simulink library "SDTlibV1"  (R2025b)
settings: Solver=VariableStepAuto  StartTime=0.0  StopTime=10.0  RelTol=1e-3
PreLoadFcn:
  | addpath(genpath('SDTfct'));
values from neighbouring files (symbols this model uses):
  pass = ra2DCMi(blk.ra)    [view_SDTlib_model.m]
undefined symbols (not defined in the file or in its folder): CMG, DAP0, DPa0, FSM, Ignew, InvDyn, InvDynAug, Jr, KIN, kinematic_model, LS, Mdyn, mnew, mp, OGnew, PMA, ra_norm, RWS, sig4, uls, ureal, uss, uw, XI
libraries: RCTblocks x470, $bdroot x4
(part 2 of 10)

== system SDTlibV1/6 dof mechanisms ==
  1 port spinning wheel : Subsystem  mask(One-port spinning wheel (6x18)){ra=[0;0;1], m=0.5, Iw=1, Ir=1/2, OG=[0;0;1], OP=[0;0;0], Omega=ureal('Omega',1000,'Range',[0 2000])}
      mask prompts: ra "Wheel axis (3x1 vector)"; m "Wheel mass (Kg)"; Iw "Wheel axial Inertia  (at G, Kgm^2)"; Ir "Wheel radial inertia (at G, Kgm^2)"; OG "OG (3x1 vector, m)"; OP "OP (3x1 vector, m)"; Omega "spinning rate (rd/s)"
      mask help:
      | Dynamic model of an onboard angular momentum (spinning wheel) at point P (connection point with a parent body):
      | 6x18 transfer between motion vector  at P and wrench applied by this body at P.
      | 0: the reference point
      | G: the center of the wheel
      | P: the connection point
      |
      | All parameters are expressed in the (inherit) body frame.
      | Only the spinning rate can be an uncertain parameter declared with "ureal"
      mask init:
      | pass=ra2DCMi(ra);
      | Tau_GP=kinematic_model(OG,OP);
      mask Help: web('DocMomentum.html','-browser','-browser')
      mask DialogControl ParameterGroupVar Prompt: Main parameters
      mask Display:
      | disp('One-port\n angular momemtum\n (6x18)')
      | port_label('input', 1, 'm')
      | port_label('output', 1, 'Wbody/.')
  2 phase stepper motor (r): TITOP model : Subsystem  mask(Stepper motor (in the load frame)){ra=[0;-1;0], z=90, p=4, n=8, I=0.17, Jr=1.1e-4, Km=4.44, C0=13e-4}
      mask prompts: ra "Direction of the joint in the local frame (3x1 vector)"; z "Rotor teeth number (integer)"; p "Stator beat number (integer)"; n "Subdivision number (integer)"; I "Current amplititude (A)"; Jr "Rotor inertia (Kg m^2)"; Km "Motor torque constant (Nm/A/rd)"; C0 "Viscous damping (Nms/rd)"
      mask help:
      | This block implement the TITOP model of a 2 phase stepper motor.
      | The direction of the revolute joint (3x1 vector) is respect with the load frame.
      |
      | LINEAR MODEL: valid around  the initial angular configuration
      | (joint angle in rad).
      |
      | Rotor inertia cannot be 0.
      mask init:
      | gam=2*pi/p/n;
      | K0=Km*I*z;
      | ra=[ra(1);ra(2);ra(3)]/norm(ra);
      | pass=[null(ra') ra];
      mask Help: web('DocStepperMotor_joly.html','-browser','-browser')
      mask Display:
      | disp('Stepper motor\n TITOP model')
      | port_label('input', 1, 'W./r')
      | port_label('output', 1, 'm_out')
      | port_label('input', 2, 'm_in')
      | port_label('output', 2, 'Wr/.')
      | port_label('input', 3, '\mu-step (int)','interpreter','tex')
      | port_label('output', 3, 'm_\theta','interpreter','tex')
  Gear box (G): TITOP model TO BE CHECKED!! : Subsystem  mask(Gear box){ra=[0;-1;0], N=-184, Jo=0.0001, Ji=0, Kg=9600, Cg=0.1}
      mask prompts: ra "Direction of the joint in the local frame (3x1 vector)"; N "Gear Box ratio"; Jo "Output shaft inertia (Kg.m^2)"; Ji "Input shaft inerta (Kg.m^2)"; Kg "Stiffness (output shaft Nm/rd)"; Cg "Viscous damping (output shaft Nms/rd)"
      mask help:
      | This block implement the TITOP model of a co-axial gearbox.
      | The direction of the gearbox axis (3x1 vector) is respect with the load frame)
      |
      | LINEAR MODEL: valid around delta_theta_o=0
      | (delta_theta_o is the geabox deflection in rad, seen from the output shaft).
      |
      | Output shaft inertia cannot be 0. If unknown, It is recommended to enter a small value (1/1000) w.r.t. the load (Kgm^2) connected on the output port.
      mask init:
      | ra=[ra(1);ra(2);ra(3)]/norm(ra);
      | pass=[null(ra') ra];
      mask Help: web('DocGearBox_joly.html','-browser','-browser')
      mask Display:
      | disp('Gear Box\n TITOP model')
      | port_label('input', 1, 'W./Go')
      | port_label('output', 1, 'm_out')
      | port_label('input', 2, 'm_in')
      | port_label('output', 2, 'WGi/.')
      | port_label('input', 3, 'Harm. pert. (Nm)')
      | port_label('output', 3, 'm_{\theta_o}','interpreter','tex')
  "Local Spring-Damper system " : Subsystem  mask(Local stiffness damper){K_O=diag([1 1 1 2 2 2]), D_O=diag([10 10 10 20 20 20]), OP=[0;0;0], OC=[0;0;0]}
      mask prompts: K_O "6x6 stiffness matrix at point O (N/m, Nm/rad)"; D_O "6x6 damping matrix  at point O (Ns/m, Nms/rad)"; OP "OP (3x1 vector (m)"; OC "OC (3x1 vector  (m)"
      mask help:
      | 12x36 TITOP model of a massless spring-damper system between:
      |   * the 2 motion vectors (inputs)  at the parent port (point P) and the child port (point C).
      |   *  the outside wrench applied to the spring-damper  at point C and the wrench applied by the spring-damper to outside at point P.
      | The model is expressed In the inherit reference frame.
      |
      | All the parameters can be declared as uncertain parameters (ureal(...)).
      mask init:
      | TAU_OC=kinematic_model([0;0;0],OC);
      | TAU_OP=kinematic_model([0;0;0],OP);
      mask Help: web('Doc_6DOFs_spring_damper.html','-browser','-browser')
      mask DialogControl ParameterGroupVar Prompt: Main parameters
      mask Display:
      | disp('Local\n spring-damper\n')
      | 
      | port_label('input', 1,'m_C')
      | port_label('output',1,'W./s,C')
      | port_label('input', 2,'m_P')
      | port_label('output',2,'Ws/.,P')
  PMA : Subsystem  mask(Proof mass actuator){Mc=0.5, IatG=diag([5e-3;5e-3;1.6e-4]), OG=[0;0;0.05], OP=[0;0;0], v=[0;0;1], mp=0.1, k=10, d=1.4}
      mask prompts: Mc "PMA total mass (Kg)"; IatG "PMA total inertia at G (Kgm^2)"; OG "OG (3x1 vector, m)"; OP "OP (3x1 vector, m)"; v "v (3x1 vector)"; mp "Proof mass (Kg)"; k "Stiffness (N/m)"; d "Damper (Ns/m)"
      mask help:
      | 7x19 dynamic model of PMA (Proof Mass Actuator) located at point P (connection point with the hub):
      |   * 6x18 transfer between motion vector at P (Xddoy,P) and wrench applied by the PMA at P (W_body/.,P).
      |   * 1 additional input: the control signal or force (N) applied to the proof mass (u_PMA),
      |   * 1 additional output: the relative position of the proof mass ./. the caging (x_PMA).
      | The model is expressed in the (inherit) body frame.
      |
      | O: refrence point
      | G: CoM of the caging,
      | P: connection point with the parent body
      |
      | v: the direction vector of the spring-mass system.
      | Each parameter (except v) can be an uncertain parameter declared with "ureal"
      mask init:
      | PG=OG-OP;
      mask Help: web('docPMA.html','-browser','-browser')
      mask Display:
      | disp('Proof Mass Actuator \n model(7x19)')
      | port_label('input', 1, 'm_P')
      | port_label('output', 1, 'Wbody/.,P')
      | port_label('input', 2, 'u_PMA')
      | port_label('output', 2, 'x_PMA')
  Prismatic joint + configuration : Subsystem  mask(Prismatic joint){ta=[1;0;0], mp=2, x=ureal('Delta',1,'range',[0.5 1.5])}
      mask prompts: ta "Direction of the joint in the local frame (3x1 vector)"; mp "Output slider mass (kg)"; x "Linear configuration (m)"
      mask help:
      | This block implement the TITOP model of a prismatic joint.
      | The last channel is the transfer between the force applied inside the joint by the input slider to the output slider and the relative linearr acceleration of the output slider w.r.t the input slider.
      |
      | Linear configuration can be a vayring parameter: Ex:
      | ureal('NAME',0,'Range',[-0.2 0.2])
      mask init:
      | pass=ra2DCMi(ta);
      | tatilde=[ta(1);ta(2);ta(3)]/norm(ta);
      | tau_x=kinematic_model(x*tatilde,[0;0;0]);
      mask Help: web('DocPrismatixJoint.html','-browser','-browser')
      mask Display:
      | disp('Prismatic joint\nTITOP model\n+ linear configuration')
      | port_label('input', 1, 'W./p,P')
      | port_label('output', 1, 'm_P')
      | port_label('input', 2, 'm_P0')
      | port_label('output', 2, 'Wp/.,P0')
      | port_label('input', 3, 'Fm')
      | port_label('output', 3, 'm_x','interpreter','tex')
  RW : Subsystem  mask(Actuated reaction wheel (7x19)){ra=[0;0;1], m=1, Iw=0.1, Ir=0.05, OG=[0;0;0], OP=[0;0;0], Omega=100}
      mask prompts: ra "Wheel axis (3x1 vector)"; m "Wheel mass (Kg)"; Iw "Wheel axial Inertia  (at G, Kgm^2)"; Ir "Wheel radial inertia (at G, Kgm^2)"; OG "OG (3x1 vector, m)"; OP "OP (3x1 vector, m)"; Omega "spinning rate (rd/s)"
      mask help:
      | Dynamic model of a reaction wheel (spinning wheel) at point P (connection point with a parent body):
      | 7x19 transfer from:
      |  * the motion vector at P (18 components)
      |  * the control signal u (Nm) : -u  is applied on the wheel along its spinning axis
      | to:
      |  * the wrench applied by this body at P (6 components).
      |  * the wheel angular acceleration.
      |
      | 0: the reference point
      | G: the center of the wheel
      | P: the connection point
      |
      | All parameters are expressed in the (inherit) body frame.
      | Only the spinning rate can be an uncertain parameter declared with "ureal"
      mask init:
      | pass=ra2DCMi(ra);
      | Tau_GP=kinematic_model(OG,OP);
      mask Help: web('DocRW.html','-browser','-browser')
      mask DialogControl ParameterGroupVar Prompt: Main parameters
      mask Display:
      | disp('Reaction wheel\n (7x19)')
      | port_label('input', 1, 'm')
      | port_label('input',2,'u (Nm)')
      | port_label('output', 1, 'Wbody/.')
      | port_label('output',2,'\Omega dot (rad/s^2)','interpreter','tex')
  RW dist : Subsystem  mask(Actuated/Disturbed reaction wheel (7x24)){ra=[0;0;1], m=1, Iw=0.1, Ir=0.05, OG=[0;0;0], OP=[0;0;0], Omega=1000}
      mask prompts: ra "Wheel axis (3x1 vector)"; m "Wheel mass (Kg)"; Iw "Wheel axial Inertia  (at G, Kgm^2)"; Ir "Wheel radial inertia (at G, Kgm^2)"; OG "OG (3x1 vector, m)"; OP "OP (3x1 vector, m)"; Omega "spinning rate (rd/s)"
      mask help:
      | Dynamic model of a reaction wheel (spinning wheel) at point P (connection point with a parent body):
      | 24x7 transfer from:
      |  * the motion vector at P (18 components)
      |  * the 5 components (3 forces, 2 radial torques) of the wheel induced disturbances (N, Nm)
      |  * the control signal u (Nm) : -u  is applied on the wheel along its spinning axis
      | to:
      |  * the wrench applied by this body at P (6 components).
      |  * the wheel angular acceleration.
      |
      | 0: the reference point
      | G: the center of the wheel
      | P: the connection point
      |
      | All parameters are expressed in the (inherit) body frame.
      | WARNING: the disturbance (input #2) is expressed in the wheel frame.
      | Only the spinning rate can be an uncertain parameter declared with "ureal"
      mask init:
      | pass=ra2DCMi(ra);
      | Tau_GP=kinematic_model(OG,OP);
      mask Help: web('DocRWdist.html','-browser','-browser')
      mask DialogControl ParameterGroupVar Prompt: Main parameters
      mask Display:
      | disp('Reaction wheel\n (7x24)')
      | port_label('input', 1, 'm')
      | port_label('input',2,'Dist: (N,Nm)')
      | port_label('input',3,'u (Nm)')
      | port_label('output', 1, 'Wbody/.')
      | port_label('output',2,'\Omega dot (rad/s^2)','interpreter','tex')
  RW_NL : Subsystem  mask(Quaqsi non-linear model of a reaction wheel (7x19)){ra=[0;0;1], m=1, Iw=0.1, Ir=0.05, OG=[0;0;0], OP=[0;0;0], Omega=1000}
      mask prompts: ra "Wheel axis (3x1 vector)"; m "Wheel mass (Kg)"; Iw "Wheel axial Inertia  (at G, Kgm^2)"; Ir "Wheel radial inertia (at G, Kgm^2)"; OG "OG (3x1 vector, m)"; OP "OP (3x1 vector, m)"; Omega "spinning rate (rd/s)"
      mask help:
      | Dynamic model of a reaction wheel (spinning wheel) at point P (connection point with a parent body):
      | 7x19 transfer from:
      |  * the motion vector at P (18 components)
      |  * the control signal u (Nm) : -u  is applied on the wheel along its spinning axis
      | to:
      |  * the wrench applied by this body at P (6 components).
      |  * the wheel spnning rate.
      |
      | 0: the reference point
      | G: the center of the wheel
      | P: the connection point
      |
      | All parameters are expressed in the (inherit) body frame.
      mask init:
      | pass=ra2DCMi(ra);
      | Tau_GP=kinematic_model(OG,OP);
      mask Help: web('DocRWnl.html','-browser','-browser')
      mask DialogControl ParameterGroupVar Prompt: Main parameters
      mask Display:
      | disp('Reaction wheel\n (7x19, NL)')
      | port_label('input', 1, 'm')
      | port_label('input',2,'u (Nm)')
      | port_label('output', 1, 'Wbody/.')
      | port_label('output',2,'\Omega (rad/s)','interpreter','tex')
  Revolute joint : Subsystem  mask(Revolute joint){ra=[0;-1;0], Jr=0.001}
      mask prompts: ra "Direction of the joint in the local frame (3x1 vector)"; Jr "Output shaft inertia (Kg m^2)"
      mask help:
      | This block implements the TITOP model of of a revolute joint.
      | The last channel is the transfer between the torque applied inside the joint by the input shaft to the output shaft and the relative angular acceleration of the output shaft w.r.t the input shaft.
      |
      | Output shaft inertia cannot be 0. If unknown, It is recommended to enter a small value (1/1000) w.r.t. the load (Kgm^2) connected on the output port.
      mask init:
      | pass=ra2DCMi(ra);
      | ran=[ra(1);ra(2);ra(3)]/norm(ra);
      mask Help: web('DocRevoluteJoint_joly.html','-browser','-browser')
      mask Display:
      | disp('Revolute joint\n TITOP model')
      | port_label('input', 1, 'W./r_out')
      | port_label('output', 1, 'm_out')
      | port_label('input', 2, 'm_in')
      | port_label('output', 2, 'Wr_in/.')
      | port_label('input', 3, 'Cm')
      | port_label('output', 3, 'm_\theta','interpreter','tex')
  Revolute joint + configuration : Subsystem  mask(Revolute joint){ra=[1;0;0], Jr=1e-9, theta=0}
      mask prompts: ra "Direction of the joint in the local frame (3x1 vector)"; Jr "Rotor inertia (kg.m^2)"; theta "Angular configuration (rad)"
      mask help:
      | This block implement the TITOP model of of a revolute joint.
      | The last channel is the transfer between the torque applied inside the joint by the input shaft to the output shaft and the relative angular acceleration of the output shaft w.r.t the input shaft.
      |
      | Angular configuration can be a vayring parameter: Ex:
      | ureal('NAME',0,'Range',[-pi pi])
      |
      | Then, ULINEARIZE will provide a model involving the block named "tan_NAME_div4";
      mask init:
      | pass=ra2DCMi(ra);
      | ran=[ra(1);ra(2);ra(3)]/norm(ra);
      mask Help: web('DocRevoluteJoint_configuration.html','-browser','-browser')
      mask Display:
      | disp('Revolute joint\nTITOP model\n+ angle configuration')
      | port_label('input', 1, 'W./r_out|a')
      | port_label('output', 1, 'm_out|a')
      | port_label('input', 2, 'm_in|p')
      | port_label('output', 2, 'Wr_in/.|p')
      | port_label('input', 3, 'Cm')
      | port_label('output', 3, 'm_\theta','interpreter','tex')
  u_sloshing : Subsystem  mask(Sloshing 1D mass-spring model(6x18)){v=[1;0;0], xi=0.001, w=0.8, m=ureal('m_slosh',5,'percent',20)}
      mask prompts: v "v (3x1 vector)"; xi "Damping ratio"; w "Frequency (rd/s)"; m "Sloshing mass attached to the spring  (kg)"
      mask help:
      | Simplified dynamic model of lateral sloshing with a spring-mass model located at point P (connection point with the hub):
      | 6x18 transfer between the motion vector at P and the wrench applied by the spring-mass system at P. The model is expressed in the (inherit) body frame.
      |
      | v: the direction vector of the spring-mass system.
      | Each parameter (except v) can be an uncertain parameter declared with "ureal"
      mask init:
      | pass=ra2DCMi(v);
      mask Help: web('Docsloshing.html','-browser','-browser')
      mask DialogControl ParameterGroupVar Prompt: Main parameters
      mask DialogControl damping Prompt: Damping ratio
      mask DialogControl mode1 Prompt: Flexible mode:
      mask Display:
      | disp('Sloshing 1D \n mass-spring \n model(6x18)')
      | port_label('input', 1, 'm')
      | port_label('output', 1, 'Wbody/.')

== system SDTlibV1/Predefined subsystems ==
  1 port flexible body + revolute joint : Subsystem  mask(One-port flexibe body with revolute joint (9x19)){m=50, Ig=[80 0 -0.1;0 20 22;-0.1 22 100], OG=[0;-2;0.03], OP=[0;0;0], ra=[0;-1;0], theta=ureal('THETA',0,'Range',[-pi pi]), n=3, xi=0.003, w1=ureal('w_SA_1',0.4*2*pi,'percent',20), L11=-0.002, L12=-1.5, L13=-5, L14=14, L15=0.02, L16=-0.01, w2=0.6*2*pi, L21=5, L22=1., L23=-0.1, L24=0., L25=2, L26=15, w3=1.5*2*pi, L31=0.3, L32=0.002, L33=0.03, L34=-0.02, L35=3.2, L36=-0.2, w4=2.83*2*pi, L41=0.0004, L42=-0.9132, L43=2.7900, L44=-1.8763, L45=-0.0246, L46=0.0031, w5=4.30*2*pi, L51=-0.0053, L52=5.878, L53=-1.0144, L54=3.0180, L55=-0.0124, L56=-0.0001, w6=0, L61=0, L62=0, L63=0, L64=0, L65=0, L66=0, w7=0, L71=0, L72=0, L73=0, L74=0, L75=0, L76=0, w8=0, L81=0, L82=0, L83=0, L84=0, L85=0, L86=0, w9=0, L91=0, L92=0, L93=0, L94=0, L95=0, L96=0, w10=0, L101=0, L102=0, L103=0, L104=0, L105=0, L106=0}
      mask prompts: m "Mass (Kg)"; Ig "Inertia (at G in Ra, Kgm^2)"; OG "OG (3x1 vector in Ra, m)"; OP "OP (3x1 vector in Ra, m)"; ra "ra (joint axis) (3x1 vector)"; theta "Angular configuration (rad)"; n "Number of flexible modes"; xi "Common damping ratio"; w1 "Frequency (rd/s)"; L11 "Tx (Kg^0.5)"; L12 "Ty (Kg^0.5)"; L13 "Tz (Kg^0.5)"; L14 "Rx (m.Kg^0.5)"; L15 "Ry (m.Kg^0.5)"; L16 "Rz (m.Kg^0.5)"; w2 "Frequency (rd/s)"; L21 "Tx (Kg^0.5)"; L22 "Ty (Kg^0.5)"; L23 "Tz (Kg^0.5)"; L24 "Rx (m.Kg^0.5)"; L25 "Ry (m.Kg^0.5)"; L26 "Rz (m.Kg^0.5)"; w3 "Frequency (rd/s)"; L31 "Tx (Kg^0.5)"; L32 "Ty (Kg^0.5)"; L33 "Tz (Kg^0.5)"; L34 "Rx (m.Kg^0.5)"; L35 "Ry (m.Kg^0.5)"; L36 "Rz (m.Kg^0.5)"; w4 "Frequency (rd/s)"; L41 "Tx (Kg^0.5)"; L42 "Ty (Kg^0.5)"; L43 "Tz (Kg^0.5)"; L44 "Rx (m.Kg^0.5)"; L45 "Ry (m.Kg^0.5)"; L46 "Rz (m.Kg^0.5)"; w5 "Frequency (rd/s)"; L51 "Tx (Kg^0.5)"; L52 "Ty (Kg^0.5)"; L53 "Tz (Kg^0.5)"; L54 "Rx (m.Kg^0.5)"; L55 "Ry (m.Kg^0.5)"; L56 "Rz (m.Kg^0.5)"; w6 "Frequency (rd/s)"; L61 "Tx (Kg^0.5)"; L62 "Ty (Kg^0.5)"; L63 "Tz (Kg^0.5)"; L64 "Rx (m.Kg^0.5)"; L65 "Ry (m.Kg^0.5)"; L66 "Rz (m.Kg^0.5)"; w7 "Frequency (rd/s)"; L71 "Tx (Kg^0.5)"; L72 "Ty (Kg^0.5)"; L73 "Tz (Kg^0.5)"; L74 "Rx (m.Kg^0.5)"; L75 "Ry (m.Kg^0.5)"; L76 "Rz (m.Kg^0.5)"; w8 "Frequency (rd/s)"; L81 "Tx (Kg^0.5)"; L82 "Ty (Kg^0.5)"; L83 "Tz (Kg^0.5)"; L84 "Rx (m.Kg^0.5)"; L85 "Ry (m.Kg^0.5)"; L86 "Rz (m.Kg^0.5)"; w9 "Frequency (rd/s)"; L91 "Tx (Kg^0.5)"; L92 "Ty (Kg^0.5)"; L93 "Tz (Kg^0.5)"; L94 "Rx (m.Kg^0.5)"; L95 "Ry (m.Kg^0.5)"; L96 "Rz (m.Kg^0.5)"; w10 "Frequency (rd/s)"; L101 "Tx (Kg^0.5)"; L102 "Ty (Kg^0.5)"; L103 "Tz (Kg^0.5)"; L104 "Rx (m.Kg^0.5)"; L105 "Ry (m.Kg^0.5)"; L106 "Rz (m.Kg^0.5)"
      mask help:
      | 9x19 dynamic model of a flexible body connected at point P to a parent body through a revolute joint:
      |  - 6x18 transfer from the motion vectort to the wrench applied by this body to the parent body at point P and
      |    projected in the parent body frame Rp.
      |  - the 3x1 channel  is the transfer:
      |               * from  the  joint torque applied by the input (parent) shaft to the output (body) shaft
      |               * to the relative motion vector of the output shaft w.r.t the input shaft [thetaddot;thetadot;theta].
      |
      | O: the body reference point
      | G: the center of mass
      | P: the connection point with a revolute joint
      | ra: direction of the revolute joint in the parent body frame Rp (or the flexible body frame Ra)
      |
      | All mechanical parameters are expressed in the flexible body frame Ra.
      | Each parameter can be an uncertain parameter declared with "ureal" (except ra)
      |
      | Angular configuration can be a vayring parameter: Ex:
      | ureal('NAME',0,'Range',[-pi pi])
      | Then, ULINEARIZE will provide a model involving the block named "tan_NAME_div4".
      mask init:
      | FlexBodyRev1Port
      mask Help: web('Doconeportflexrevolute.html','-browser','-browser')
      mask TypeOptions n: 0 | 1 | 2 | 3 | 4 | 5 | 6 | 7 | 8 | 9 | 10
      mask DialogControl ParameterGroupVar Prompt: Main parameters
      mask DialogControl damping Prompt: Damping ratio
      mask DialogControl mode1 Prompt: Flexible mode #1:
      mask DialogControl Control8 Prompt: Modal participation factor at P in Ra
      mask DialogControl mode2 Prompt: #2:
      mask DialogControl Control9 Prompt: Modal participation factor at P in Ra
      mask DialogControl mode3 Prompt: #3
      mask DialogControl Control10 Prompt: Modal participation factor at P in Ra
      mask DialogControl mode4 Prompt: #4
      mask DialogControl Control11 Prompt: Modal participation factor at P in Ra
      mask DialogControl mode5 Prompt: #5
      mask DialogControl Control12 Prompt: Modal participation factor at P in Ra
      mask DialogControl mode6 Prompt: #6
      mask DialogControl Control13 Prompt: Modal participation factor at P in Ra
      mask DialogControl mode7 Prompt: #7
      mask DialogControl Control14 Prompt: Modal participation factor at P in Ra
      mask DialogControl mode8 Prompt: #8
      mask DialogControl Control15 Prompt: Modal participation factor at P in Ra
      mask DialogControl mode9 Prompt: #9
      mask DialogControl Control16 Prompt: Modal participation factor at P in Ra
      mask DialogControl mode10 Prompt: #10
      mask DialogControl Control17 Prompt: Modal participation factor at P in Ra
      mask Display:
      | disp('One-port\n flexible body\n + revolute joint\n (9x19)')
      | port_label('input', 1, 'm')
      | port_label('output', 1, 'Wbody/.')
      | port_label('input', 2, 'Cm')
      | port_label('output', 2, 'm_\theta','interpreter','tex')
  Multi port rigid body + prismatic joint : Subsystem  mask(Multi-port rigid body with prismatic joint (18n-9)x(6n+13)){m=100, Ig=[20 0 0; 0 20 0; 0 0 20], OG=[0;0;0], n=3, OP1=[0;0;0], OP2=[0;0;0], OP3=[0;0;0], OP4=[0;0;1], OP5=[0;0;0], ta=[0;-1;0], x=ureal('x',0,'Range',[-0.5 0.5])}
      mask prompts: m "Mass (kg)"; Ig "Inertia at G in Ra (kg.m^2)"; OG "OG (3x1 vector in Ra)  (m)"; n "n (number of connection points)"; OP1 "OP1 (3x1 vector in Ra) (m)"; OP2 "OP2 (3x1 vector in Ra) (m)"; OP3 "OP3 (3x1 vector in Ra) (m)"; OP4 "OP4 (3x1 vector in Ra) (m)"; OP5 "OP5 (3x1 vector in Ra) (m)"; ta "ta (joint axis) (3x1 vector)"; x "Linear configuration (m)"
      mask help:
      | Computes the (18n-9)x(6n+13) model :
      | - 6x18 transfer from the motion vector to the wrench applied by this body to a parent body at port P1 through a prismatic joint
      | - the 3x1 channel :
      |               * from  the  joint force applied by the input (parent) slider to the output (body) slider
      |               * to the relative motion vector of the output slider w.r.t the input slider ([xddot;xdot;x]).
      | - (n-1) 18x6 transfers from the wrenches applied to this body to the motion vectors at ports P2,P3,..,
      |
      | Input/Output of port P1 are expressed w.r.t; point P10 (P1 coincides with P10 when the linear configuration is null)
      |
      | O: the body reference point
      | G: the center of mass
      | Pi (i=1:n): the n given connection points or ports (n<6).
      | ta: direction of the prismatic joint in the inherit frame Rp (or the body framer Ra)
      | x: linear configuration of the joint (P1 is obtained from P10 by a translation of x along ta).
      |
      | All parameters must be expressed in the body frame Ra=Rp.
      | Each parameter can be an uncertain parameter declared with the function ureal (except ta)
      mask init:
      | MultiPortRigidBodyPrisAug
      mask Help: web('DocMultiportRigidBodyPrismatic.html','-browser','-browser')
      mask TypeOptions n: 1 | 2 | 3 | 4 | 5
      mask DialogControl ParameterGroupVar Prompt: Rigid body parameter
      mask DialogControl port1 Prompt: #1
      mask DialogControl port2 Prompt: #2
      mask DialogControl port3 Prompt: #3
      mask DialogControl port4 Prompt: #4
      mask DialogControl port5 Prompt: #5
      mask DialogControl JointParameters Prompt: Prismatic joint parameters
      mask Display:
      | disp('Multi-port\n rigid body\n+ prismatic joint \n(18n-9)x(6n+13)')
      | 
      | port_label('input', 1,'m_P10')
      | port_label('output',1,'Wbody/.,P10')
      | port_label('input', 2,'Fm_at_P1')
      | port_label('output',2,'m_x at P1','interpreter','tex')
      | 
      | if n>1
      |     for i=2:n
      |         port_label('input', i+1,['W./body,P',num2str(i)])
      |         port_label('output',i+1,['m_P',num2str(i)])
      |     end
      | end
  Multi port rigid body + revolute joint : Subsystem  mask(Multi-port rigid body with revolute joint (18n-9)x(6n+15)){m=60, Ig=[1.6 0 0; 0 1.6 0; 0 0 0.67], OG=[0;0;0.25], n=3, OP1=[0;0;0], OP2=[0;0;0.5], OP3=[0;0;0.25], OP4=[0;12;0], OP5=[0;0;0], ra=[0;0;1], theta=ureal('theta1',0,'Range',[-pi pi])}
      mask prompts: m "Mass (kg)"; Ig "Inertia at G in Ra (kg.m^2)"; OG "OG (3x1 vector in Ra)  (m)"; n "n (number of connection points)"; OP1 "OP1 (3x1 vector in Ra) (m)"; OP2 "OP2 (3x1 vector in Ra) (m)"; OP3 "OP3 (3x1 vector in Ra) (m)"; OP4 "OP4 (3x1 vector in Ra) (m)"; OP5 "OP5 (3x1 vector in Ra) (m)"; ra "ra (joint axis) (3x1 vector)"; theta "Angular configuration (rad)"
      mask help:
      | Computes the (18n-9)x(6n+13) model :
      | - 6x18 transfer from the motion vector to the wrench applied by this body to a parent body at port P1 through a revolute joint,
      | - the 3x1 channel :
      |               * from  the  joint torque applied by the input (parent) shaft to the output (body) shaft
      |               * to the relative motion vector of the output shaft w.r.t the input shaft ([thetaddot;thetadot;theta]),
      | - (n-1) 18x6 transfers from the wrenches applied to this body to the motion vectors at ports P2,P3,..,
      |
      | Input/Output of port P1 are expressed in the parent frame Rp
      | Input/Output of ports P2,P3,... are expressed in the body frame Ra.
      |
      | O: the body reference point
      | G: the center of mass
      | Pi (i=1:n): the n given connection points or ports (n<6).
      | ra: direction of the revolute joint in the Rp (or Ra)
      | theta: angular configuration of the joint (Ra is obtained from Rp by a rotation of theta around ra).
      |
      | All parameters must be expressed in the body frame Ra.
      | Each parameter can be an uncertain parameter declared with the function ureal (except ra)
      |
      | Rk: if "theta" field is: ureal('NAME',0,'Range',[-pi pi])
      | then, ULINEARIZE will provide a model involving the block named "tan_NAME_div4";
      mask init:
      | MultiPortRigidBodyRevAug
      mask Help: web('DocMultiportRigidBodyRevolute.html','-browser','-browser')
      mask TypeOptions n: 1 | 2 | 3 | 4 | 5
      mask DialogControl ParameterGroupVar Prompt: Rigid body parameter
      mask DialogControl port1 Prompt: #1
      mask DialogControl port2 Prompt: #2
      mask DialogControl port3 Prompt: #3
      mask DialogControl port4 Prompt: #4
      mask DialogControl port5 Prompt: #5
      mask DialogControl JointParameters Prompt: Revolute joint parameters
      mask Display:
      | disp('Multi-port\n rigid body\n+ revolute joint \n(18n-9)x(6n+13)')
      | 
      | port_label('input', 1,'m_P1|p')
      | port_label('output',1,'Wbody/.,P1|p')
      | port_label('input', 2,'Cm_at_P1')
      | port_label('output',2,'m_\theta at P1','interpreter','tex')
      | 
      | if n>1
      |     for i=2:n
      |         port_label('input', i+1,['W./body,P',num2str(i),'|a'])
      |         port_label('output',i+1,['m_P',num2str(i),'|a'])
      |     end
      | end
  TITOP flexible beam +revolute joint : Subsystem  mask(TITOP flexible beam with revolute joint (27x25)){l=6.4, s=2*pi*0.01*0.1, rho=2700, E=70e9, Iz=pi*(0.105^4-0.095^4)/4, Iy=pi*(0.105^4-0.095^4)/4, ni=0.35, xi=0.001, Won=off, uw_var=10, Nflex=3, ra=[0;-1;0], theta=ureal('theta',0,'Range',[-pi pi])}
      mask prompts: l "length along x (m)"; s "cross section (m^2)"; rho "mass density (Kg/m^3)"; E "Young modulus (N/m^2)"; Iz "second moment of area along z axis, Iz (m^4)"; Iy "second moment of area along y axis Iy, (m^4)"; ni "Poisson coefficient"; xi "dampig ratio"; uw_var "uncertainty (d_w, %)"; Nflex "number of flexible mode (Nflex, integer<=10)"; ra "ra (joint axis) (3x1 vector)"; theta "angular configuration (rad)"
      mask help:
      | Computes the 27x25 model :
      | - 18x6 transfer from the wrenches applied to this body to the motion vector at port C,
      | - the 3x1 channel:
      |               * from  the  joint torque applied by the input (parent) shaft to the output (body) shaft
      |               * to the relative motion vector of the output shaft w.r.t the input shaft [thetaddot;thetadot;theta].
      | - 6x18 transfer from the motion vector to the wrench applied by this body to a parent body at port P through a revolute joint
      |
      | Input/Output of port P are expressed in the parent frame Rp
      | Input/Output of port C are expressed in the body frame Ra.
      |
      | ra: direction of the revolute joint in the Rp (or Ra)
      | theta: angular configuration of the joint (Ra is obtained from Rp by a rotation of theta around ra).
      |
      | All parameters must be expressed in the body frame Ra.
      | Each parameter can be an uncertain parameter declared with the function ureal (except ra)
      |
      | Rk: if "theta" field is: ureal('NAME',0,'Range',[-pi pi])
      | then, ULINEARIZE will provide a model involving the block named "tan_NAME_div4";
      mask init:
      | BeamRev2PortAug
      mask Help: web('DocBeamRevolute.html','-browser','-browser')
      mask DialogControl Container5 Prompt: Direct uncertainties on flexible mode frequencies
      mask DialogControl Control2 Prompt: Uncertainties on physical parameters (length, mass, ..) can create huge LFTs.
      mask DialogControl Control3 Prompt: Check this box to overwrite physical parameter uncertainties by a common relative uncertainty (d_w, %) on the first (Nflex) flexible mode frequencies of the clamped at P / free at C beam.
      mask DialogControl Control4 Prompt: The uncertain frequency is named: 'w_name_i' where:
      mask DialogControl Control5 Prompt: * 'name' is the current block name (reduced to its alphanumeric characters).
      mask DialogControl Control6 Prompt: * 'i' is the flexible mode number (increasing frequency order)
      mask DialogControl Container6 Prompt: Joint data
      mask Display:
      | disp('TITOP flexible beam\n + revolute joint\n (27x25)')
      | 
      | port_label('input', 1,'W./body,C|a')
      | port_label('output',1,'m_C|a')
      | port_label('input', 2,'Cm_at_P')
      | port_label('output',2,'m_\theta at P','interpreter','tex')
      | port_label('input', 3,'m_P|p')
      | port_label('output',3,'Wbody/.,P|p')

== system SDTlibV1/Space  subsystems ==
  2 axis (x-y) Fast Steering Mirror (FSM) : Subsystem
  Four CMGs Pyramid : Subsystem
  RWS : Subsystem
  Set of 6 PMAss : Subsystem

== system SDTlibV1/Subsystem ==

== system SDTlibV1/3//6//18 DCM/18x18 DCM ==
  u : Inport  PortDimensions=18
  Demux : Demux  Outputs=[3 3 3 3 3 3]
  Mux : Mux  Inputs=[3 3 3 3 3 3]
  rotation : Gain  Gain=rot  Multiplication=Matrix(K*u) (u vector)
  rotation1 : Gain  Gain=rot  Multiplication=Matrix(K*u) (u vector)
  rotation2 : Gain  Gain=rot  Multiplication=Matrix(K*u) (u vector)
  translation : Gain  Gain=rot  Multiplication=Matrix(K*u) (u vector)
  translation1 : Gain  Gain=rot  Multiplication=Matrix(K*u) (u vector)
  translation2 : Gain  Gain=rot  Multiplication=Matrix(K*u) (u vector)
  y : Outport  VectorParamsAs1DForOutWhenUnconnected=off
  wires:
  rotation/1 -> Mux/2
  translation/1 -> Mux/1
  Demux/1 -> translation/1
  u/1 -> Demux/1
  Mux/1 -> y/1
  Demux/2 -> rotation/1
  Demux/4 -> rotation1/1
  Demux/3 -> translation1/1
  translation1/1 -> Mux/3
  rotation1/1 -> Mux/4
  Demux/5 -> translation2/1
  translation2/1 -> Mux/5
  rotation2/1 -> Mux/6
  Demux/6 -> rotation2/1

== system SDTlibV1/3//6//18 DCM/18x18 v-u_rotation ==
  u : Inport  PortDimensions=18
  Demux : Demux  Outputs=[3 3 3 3 3 3]
  Mux : Mux  Inputs=[3 3 3 3 3 3]
  Subsystem : Subsystem
  Subsystem1 : Subsystem
  Subsystem2 : Subsystem
  Subsystem3 : Subsystem
  Subsystem4 : Subsystem
  Subsystem5 : Subsystem
  y : Outport  VectorParamsAs1DForOutWhenUnconnected=off
  wires:
  Subsystem1/1(Out1) -> Mux/2
  Subsystem/1(Out1) -> Mux/1
  Demux/2 -> Subsystem1/1(In1)
  Demux/1 -> Subsystem/1(In1)
  u/1 -> Demux/1
  Mux/1 -> y/1
  Demux/3 -> Subsystem2/1(In1)
  Subsystem2/1(Out1) -> Mux/3
  Demux/4 -> Subsystem3/1(In1)
  Subsystem3/1(Out1) -> Mux/4
  Demux/5 -> Subsystem4/1(In1)
  Subsystem4/1(Out1) -> Mux/5
  Demux/6 -> Subsystem5/1(In1)
  Subsystem5/1(Out1) -> Mux/6

== system SDTlibV1/3//6//18 DCM/3x3 v-u_rotation ==
  u : Inport  PortDimensions=3
  Demux : Demux  Outputs=3
  Gain : Gain  Gain=2
  Gain1 : Gain  Gain=-2
  Gain2 : Gain  Gain=2
  Gain3 : Gain  Gain=2
  Gain4 : Gain  Gain=pass  Multiplication=Matrix(K*u) (u vector)
  Gain5 : Gain  Gain=pass'  Multiplication=Matrix(K*u) (u vector)
  Mux : Mux  Inputs=3
  Sum : Sum  Inputs=++|
  Sum1 : Sum  Inputs=|++
  Sum2 : Sum  Inputs=|+-
  Sum3 : Sum  Inputs=|++
  Sum4 : Sum  Inputs=++|
  Sum5 : Sum  Inputs=++|
  Uncertain State Space{,1..3} (4 alike) : RCTblocks/Uncertain State Space  Tag=USS  USystem=uss(sig4)  UValue=[]  X0=[]  uX0=[]
  y : Outport  VectorParamsAs1DForOutWhenUnconnected=off
  wires:
  Demux/3 -> Mux/3
  Sum5/1 -> Gain2/1
  Uncertain State Space2/1 -> Uncertain State Space3/1, Sum4/2, Sum2/2
  Sum/1 -> Uncertain State Space/1
  Sum3/1 -> Uncertain State Space2/1
  Uncertain State Space/1 -> Uncertain State Space1/1, Sum5/1, Sum1/1
  Uncertain State Space1/1 -> Sum/1
  Gain3/1 -> Sum5/2
  Gain2/1 -> Sum3/1
  Demux/1 -> Gain3/1, Sum1/2
  Mux/1 -> Gain4/1
  Uncertain State Space3/1 -> Sum3/2
  Sum1/1 -> Mux/1
  Gain/1 -> Sum/2
  Demux/2 -> Sum4/1, Gain1/1
  Sum4/1 -> Mux/2
  Gain1/1 -> Sum2/1
  Sum2/1 -> Gain/1
  Gain4/1 -> y/1
  Gain5/1 -> Demux/1
  u/1 -> Gain5/1

== system SDTlibV1/3//6//18 DCM/3x3 z-u_rotation ==
  u : Inport  PortDimensions=3
  Demux : Demux  Outputs=3
  Gain : Gain  Gain=2
  Gain1 : Gain  Gain=-2
  Gain2 : Gain  Gain=2
  Gain3 : Gain  Gain=2
  Mux : Mux  Inputs=3
  Sum : Sum  Inputs=++|
  Sum1 : Sum  Inputs=|++
  Sum2 : Sum  Inputs=|+-
  Sum3 : Sum  Inputs=|++
  Sum4 : Sum  Inputs=++|
  Sum5 : Sum  Inputs=++|
  Uncertain State Space{,1..3} (4 alike) : RCTblocks/Uncertain State Space  Tag=USS  USystem=uss(sig4)  UValue=[]  X0=[]  uX0=[]
  y : Outport  VectorParamsAs1DForOutWhenUnconnected=off
  wires:
  Sum2/1 -> Gain/1
  Gain1/1 -> Sum2/1
  Sum4/1 -> Mux/2
  Demux/2 -> Sum4/1, Gain1/1
  Gain/1 -> Sum/2
  Sum1/1 -> Mux/1
  u/1 -> Demux/1
  Uncertain State Space3/1 -> Sum3/2
  Mux/1 -> y/1
  Demux/1 -> Sum1/2, Gain3/1
  Gain2/1 -> Sum3/1
  Gain3/1 -> Sum5/2
  Uncertain State Space1/1 -> Sum/1
  Uncertain State Space/1 -> Sum1/1, Sum5/1, Uncertain State Space1/1
  Sum3/1 -> Uncertain State Space2/1
  Sum/1 -> Uncertain State Space/1
  Uncertain State Space2/1 -> Sum4/2, Sum2/2, Uncertain State Space3/1
  Sum5/1 -> Gain2/1
  Demux/3 -> Mux/3

== system SDTlibV1/3//6//18 DCM/6x6 DCM ==
  u : Inport  PortDimensions=6
  Demux : Demux  Outputs=[3 3]
  Mux : Mux  Inputs=[3 3]
  rotation : Gain  Gain=rot  Multiplication=Matrix(K*u) (u vector)
  translation : Gain  Gain=rot  Multiplication=Matrix(K*u) (u vector)
  y : Outport  VectorParamsAs1DForOutWhenUnconnected=off
  wires:
  Demux/2 -> rotation/1
  Mux/1 -> y/1
  u/1 -> Demux/1
  Demux/1 -> translation/1
  translation/1 -> Mux/1
  rotation/1 -> Mux/2

== system SDTlibV1/3//6//18 DCM/6x6 v-u_rotation ==
  u : Inport  PortDimensions=6
  Demux : Demux  Outputs=[3 3]
  Mux : Mux  Inputs=[3 3]
  Subsystem : Subsystem
  Subsystem1 : Subsystem
  y : Outport  VectorParamsAs1DForOutWhenUnconnected=off
  wires:
  Mux/1 -> y/1
  u/1 -> Demux/1
  Demux/1 -> Subsystem/1(In1)
  Demux/2 -> Subsystem1/1(In1)
  Subsystem/1(Out1) -> Mux/1
  Subsystem1/1(Out1) -> Mux/2

== system SDTlibV1/3//6//18 DCM/6x6 z-u_rotation ==
  u : Inport  PortDimensions=6
  Demux : Demux  Outputs=[3 3]
  Mux : Mux  Inputs=[3 3]
  Subsystem : Subsystem
  Subsystem1 : Subsystem
  y : Outport  VectorParamsAs1DForOutWhenUnconnected=off
  wires:
  Mux/1 -> y/1
  u/1 -> Demux/1
  Demux/1 -> Subsystem/1(In1)
  Subsystem/1(Out1) -> Mux/1
  Demux/2 -> Subsystem1/1(In1)
  Subsystem1/1(Out1) -> Mux/2

== system SDTlibV1/6 dof bodies/ 2 ports flexible beam ==
  in1 : Inport  PortDimensions=6
  in2 : Inport  Port=2  PortDimensions=6
  Demux : Demux  Outputs=[18 18]
      settings: DisplayOption=none
  Mux : Mux  Inputs=[6 6]
  Uncertain State Space : RCTblocks/Uncertain State Space  Tag=USS  USystem=TITOPBEAM  UValue=[]  X0=[]  uX0=[]
  out1 : Outport  VectorParamsAs1DForOutWhenUnconnected=off
  out2 : Outport  Port=2  VectorParamsAs1DForOutWhenUnconnected=off
  wires:
  Demux/2 -> out2/1
  in2/1 -> Mux/2
  Demux/1 -> out1/1
  in1/1 -> Mux/1
  Uncertain State Space/1 -> Demux/1
  Mux/1 -> Uncertain State Space/1

== system SDTlibV1/6 dof bodies/ N ports Nastran (free) body ==
  in1 : Inport  PortDimensions=6
  in2 : Inport  Port=2  PortDimensions=6
  in3 : Inport  Port=3  PortDimensions=6
  in4 : Inport  Port=4  PortDimensions=6
  in5 : Inport  Port=5  PortDimensions=6
  Demux : Demux  Outputs=[18 18 18 18 18]
  Gain : RCTblocks/Uncertain State Space  Tag=USS  USystem=Mdyn  UValue=[]  X0=[]  uX0=[]
  Mux : Mux  Inputs=[6 6 6 6 6]
  out1 : Outport
  out2 : Outport  Port=2
  out3 : Outport  Port=3
  out4 : Outport  Port=4
  out5 : Outport  Port=5
  wires:
  Mux/1 -> Gain/1
  Gain/1 -> Demux/1
  in1/1 -> Mux/1
  Demux/1 -> out1/1
  in2/1 -> Mux/2
  Demux/2 -> out2/1
  in3/1 -> Mux/3
  Demux/3 -> out3/1
  in4/1 -> Mux/4
  Demux/4 -> out4/1
  in5/1 -> Mux/5
  Demux/5 -> out5/1

== system SDTlibV1/6 dof bodies/ N ports flexible body ==
  W_./body,C1 : Inport  PortDimensions=6
  W_./body,C2 : Inport  Port=2  PortDimensions=6
  m_P : Inport  Port=3  PortDimensions=18
  Demux : Demux  Outputs=[18 18 6]
  Gain : RCTblocks/Uncertain State Space  Tag=USS  USystem=Mdyn  UValue=[]  X0=[]  uX0=[]
  Mux : Mux  Inputs=[6 6 18]
  m_C1 : Outport
  m_C2 : Outport  Port=2
  W_body/.,P : Outport  Port=3
  wires:
  Mux/1 -> Gain/1
  Gain/1 -> Demux/1
  W_./body,C1/1 -> Mux/1
  Demux/1 -> m_C1/1
  W_./body,C2/1 -> Mux/2
  Demux/2 -> m_C2/1
  m_P/1 -> Mux/3
  Demux/3 -> W_body/.,P/1

== system SDTlibV1/6 dof bodies/1 port Nastran body ==
  m : Inport  PortDimensions=18
  2*xi diagonal matrix : RCTblocks/Uncertain State Space  Tag=USS  USystem=uss(2*XI)  UValue=[]  X0=[]  uX0=[]
  Add : Sum  Inputs=--
  Add1 : Sum
  Add2 : Sum  Inputs=+-
  DAp0 : Gain  Gain=DPa0  Multiplication=Matrix(K*u)
  Demux : Demux  Outputs=[6 12]
  Integrator : Integrator
  Integrator1 : Integrator
  Terminator : Terminator
  "[Lp] ' Ra" : Gain  Gain=LS'  Multiplication=Matrix(K*u)
  "[Lp] Ra" : Gain  Gain=LS  Multiplication=Matrix(K*u)
  omega diagonal matrix. : RCTblocks/Uncertain State Space  Tag=USS  USystem=uss(diag(uw))  UValue=[]  X0=[]  uX0=[]
  omega diagonal matrix.1 : RCTblocks/Uncertain State Space  Tag=USS  USystem=uss(diag(uw))  UValue=[]  X0=[]  uX0=[]
  Wbody/. : Outport  VectorParamsAs1DForOutWhenUnconnected=off
  wires:
  Add2/1 -> Wbody/./1  "[ Wbody/.,P]/Ra"
  Integrator1/1 -> omega diagonal matrix./1  "eta"
  "[Lp] ' Ra"/1 -> Add2/1
  Add1/1 -> omega diagonal matrix.1/1
  Add/1 -> Integrator/1  "eta dot dot"
  "[Lp] Ra"/1 -> Add/2
  omega diagonal matrix.1/1 -> Add/1, "[Lp] ' Ra"/1
  2*xi diagonal matrix/1 -> Add1/2
  DAp0/1 -> Add2/2
  Integrator/1 -> 2*xi diagonal matrix/1, Integrator1/1  "eta dot"
  omega diagonal matrix./1 -> Add1/1
  Demux/2 -> Terminator/1
  m/1 -> Demux/1
  Demux/1 -> DAp0/1, "[Lp] Ra"/1  "[ Xddot(p) ]/Ra"

== system SDTlibV1/6 dof bodies/1 port flexible body ==
  m : Inport  PortDimensions=18
  2*xi diagonal matrix : RCTblocks/Uncertain State Space  Tag=USS  USystem=uss(2*XI)  UValue=[]  X0=[]  uX0=[]
  Add : Sum  Inputs=--
  Add1 : Sum
  Add2 : Sum  Inputs=+-
  DAP0 : RCTblocks/Uncertain State Space  Tag=USS  USystem=uss(DAP0)  UValue=[]  X0=[]  uX0=[]
  Demux : Demux  Outputs=[6 12]
  Integrator : Integrator
  Integrator1 : Integrator
  Terminator : Terminator
  "[Lp] ' Ra" : RCTblocks/Uncertain State Space  Tag=USS  USystem=uss(uls')  UValue=[]  X0=[]  uX0=[]
  "[Lp] Ra" : RCTblocks/Uncertain State Space  Tag=USS  USystem=uss(uls)  UValue=[]  X0=[]  uX0=[]
  omega diagonal matrix : RCTblocks/Uncertain State Space  Tag=USS  USystem=uss(diag(uw))  UValue=[]  X0=[]  uX0=[]
  omega diagonal matrix. : RCTblocks/Uncertain State Space  Tag=USS  USystem=uss(diag(uw))  UValue=[]  X0=[]  uX0=[]
  Wbody/. : Outport  VectorParamsAs1DForOutWhenUnconnected=off
  wires:
  Demux/2 -> Terminator/1
  Demux/1 -> DAP0/1, "[Lp] Ra"/1  "[ Xddot_P]/Ra"
  m/1 -> Demux/1
  DAP0/1 -> Add2/2
  "[Lp] ' Ra"/1 -> Add2/1
  omega diagonal matrix./1 -> Add1/1
  Integrator/1 -> 2*xi diagonal matrix/1, Integrator1/1  "eta dot"
  Integrator1/1 -> omega diagonal matrix./1  "eta"
  Add/1 -> Integrator/1  "eta dot dot"
  Add1/1 -> omega diagonal matrix/1
  2*xi diagonal matrix/1 -> Add1/2
  "[Lp] Ra"/1 -> Add/2
  omega diagonal matrix/1 -> "[Lp] ' Ra"/1, Add/1
  Add2/1 -> Wbody/./1  "[ Wbody/.,P ]/Ra"

== system SDTlibV1/6 dof bodies/Multi in//out-port flexible body ==
  in1 : Inport  PortDimensions=6
  in2 : Inport  Port=2  PortDimensions=6
  in3 : Inport  Port=3  PortDimensions=6
  Demux : Demux  Outputs=[18 18 18 18]
  Gain : RCTblocks/Uncertain State Space  Tag=USS  USystem=uss(Mdyn)  UValue=[]  X0=[]  uX0=[]
  Mux : Mux  Inputs=[6 6 6]
  out1 : Outport
  out2 : Outport  Port=2
  out3 : Outport  Port=3
  out4 : Outport  Port=4
  wires:
  Mux/1 -> Gain/1
  in1/1 -> Mux/1
  in2/1 -> Mux/2
  in3/1 -> Mux/3
  Gain/1 -> Demux/1
  Demux/1 -> out1/1
  Demux/2 -> out2/1
  Demux/3 -> out3/1
  Demux/4 -> out4/1

== system SDTlibV1/6 dof bodies/Multi port flexible body ==
  in1 : Inport  PortDimensions=6
  in2 : Inport  Port=2  PortDimensions=6
  in3 : Inport  Port=3  PortDimensions=6
  in4 : Inport  Port=4  PortDimensions=18
  Demux : Demux  Outputs=[18 18 18 6]
  Gain : RCTblocks/Uncertain State Space  Tag=USS  USystem=uss(Mdyn)  UValue=[]  X0=[]  uX0=[]
  Mux : Mux  Inputs=[6 6 6 18]
  out1 : Outport
  out2 : Outport  Port=2
  out3 : Outport  Port=3
  out4 : Outport  Port=4
  wires:
  Mux/1 -> Gain/1
  Gain/1 -> Demux/1
  in1/1 -> Mux/1
  Demux/1 -> out1/1
  in2/1 -> Mux/2
  Demux/2 -> out2/1
  in3/1 -> Mux/3
  Demux/3 -> out3/1
  in4/1 -> Mux/4
  Demux/4 -> out4/1

== system SDTlibV1/6 dof bodies/Multi port rigid body ==
  in1 : Inport  PortDimensions=6
  in2 : Inport  Port=2  PortDimensions=6
  in3 : Inport  Port=3  PortDimensions=18
  Demux : Demux  Outputs=[ 18 18 6]
      settings: DisplayOption=none
  Gain : RCTblocks/Uncertain State Space  Tag=USS  USystem=uss(InvDynAug)  UValue=[]  X0=[]  uX0=[]
  Mux : Mux  Inputs=[ 6 6 18]
  out1 : Outport
  out2 : Outport  Port=2
  out3 : Outport  Port=3
  wires:
  Mux/1 -> Gain/1
  Gain/1 -> Demux/1
  in1/1 -> Mux/1
  Demux/1 -> out1/1
  in2/1 -> Mux/2
  Demux/2 -> out2/1
  in3/1 -> Mux/3
  Demux/3 -> out3/1

== system SDTlibV1/6 dof bodies/Multi port rigid free body ==
  W_./body,P1 : Inport  PortDimensions=6
  W_./body,P2 : Inport  Port=2  PortDimensions=6
  W_./body,P3 : Inport  Port=3  PortDimensions=6
  Demux : Demux  Outputs=[18 18 18]
      settings: DisplayOption=none
  Gain : RCTblocks/Uncertain State Space  Tag=USS  USystem=uss(InvDyn)  UValue=[]  X0=[]  uX0=[]
  Mux : Mux  Inputs=[6 6 6]
  m_P1 : Outport
  m_P2 : Outport  Port=2
  m_P3 : Outport  Port=3
  wires:
  Mux/1 -> Gain/1
  Gain/1 -> Demux/1
  W_./body,P1/1 -> Mux/1
  Demux/1 -> m_P1/1
  W_./body,P2/1 -> Mux/2
  Demux/2 -> m_P2/1
  W_./body,P3/1 -> Mux/3
  Demux/3 -> m_P3/1

== system SDTlibV1/6 dof bodies/massless connection body ==
  in1 : Inport  PortDimensions=6
  in2 : Inport  Port=2  PortDimensions=6
  in3 : Inport  Port=3  PortDimensions=18
  in4 : Inport  Port=4  PortDimensions=6
  Demux : Demux  Outputs=[ 18 18 6 18]
      settings: DisplayOption=none
  Gain : RCTblocks/Uncertain State Space  Tag=USS  USystem=uss(KIN)  UValue=[]  X0=[]  uX0=[]
  Mux : Mux  Inputs=[ 6 6 18 6]
  out1 : Outport  VectorParamsAs1DForOutWhenUnconnected=off
  out2 : Outport  Port=2  VectorParamsAs1DForOutWhenUnconnected=off
  out3 : Outport  Port=3  VectorParamsAs1DForOutWhenUnconnected=off
  out4 : Outport  Port=4  VectorParamsAs1DForOutWhenUnconnected=off
  wires:
  Mux/1 -> Gain/1
  Gain/1 -> Demux/1
  in1/1 -> Mux/1
  Demux/1 -> out1/1
  in2/1 -> Mux/2
  Demux/2 -> out2/1
  in3/1 -> Mux/3
  Demux/3 -> out3/1
  in4/1 -> Mux/4
  Demux/4 -> out4/1

== system SDTlibV1/6 dof bodies/multi-port FEM Kirchhoff plate ==
  in1 : Inport  PortDimensions=6
  in2 : Inport  Port=2  PortDimensions=6
  in3 : Inport  Port=3  PortDimensions=6
  in4 : Inport  Port=4  PortDimensions=18
  in5 : Inport  Port=5  PortDimensions=18
  Demux : Demux  Outputs=[18 18 18 6 6 ]
  Mux : Mux  Inputs=[6 6 6 18 18 ]
  ninop : RCTblocks/Uncertain State Space  Tag=USS  USystem=NINOP  UValue=[]  X0=[]  uX0=[]
  out1 : Outport
  out2 : Outport  Port=2
  out3 : Outport  Port=3
  out4 : Outport  Port=4
  out5 : Outport  Port=5
  wires:
  Mux/1 -> ninop/1
  ninop/1 -> Demux/1
  in1/1 -> Mux/1
  Demux/1 -> out1/1
  in2/1 -> Mux/2
  Demux/2 -> out2/1
  in3/1 -> Mux/3
  Demux/3 -> out3/1
  in4/1 -> Mux/4
  Demux/4 -> out4/1
  in5/1 -> Mux/5
  Demux/5 -> out5/1

== system SDTlibV1/6 dof bodies/multi-port flexible plate ==
  in1 : Inport  PortDimensions=6
  in2 : Inport  Port=2  PortDimensions=6
  in3 : Inport  Port=3  PortDimensions=6
  in4 : Inport  Port=4  PortDimensions=18
  Demux : Demux  Outputs=[18 18 18 6 ]
  Mux : Mux  Inputs=[6 6 6 18 ]
  ninop : RCTblocks/Uncertain State Space  Tag=USS  USystem=NINOP  UValue=[]  X0=[]  uX0=[]
  out1 : Outport
  out2 : Outport  Port=2
  out3 : Outport  Port=3
  out4 : Outport  Port=4
  wires:
  Mux/1 -> ninop/1
  ninop/1 -> Demux/1
  in1/1 -> Mux/1
  Demux/1 -> out1/1
  in2/1 -> Mux/2
  Demux/2 -> out2/1
  in3/1 -> Mux/3
  Demux/3 -> out3/1
  in4/1 -> Mux/4
  Demux/4 -> out4/1

== system SDTlibV1/6 dof mechanisms/1 port spinning wheel ==
  m : Inport  PortDimensions=18
  Demux : Demux  Outputs=[3 3]
  Demux2 : Demux  Outputs=[6 6 6]
  Demux3 : Demux  Outputs=[3 3]
  Gain1 : Gain  Gain=pass'  Multiplication=Matrix(K*u) (u vector)
  Gain10 : Gain  Gain=pass'  Multiplication=Matrix(K*u) (u vector)
  Gain2 : Gain  Gain=pass  Multiplication=Matrix(K*u) (u vector)
  Gain3 : Gain  Gain=m*eye(3)  Multiplication=Matrix(K*u) (u vector)
  Gain4 : Gain  Gain=diag([Ir Ir Iw])  Multiplication=Matrix(K*u) (u vector)
  Gain5 : Gain  Gain=[1 0 0;0 1 0]  Multiplication=Matrix(K*u) (u vector)
  Gain6 : Gain  Gain=[0 Iw;-Iw 0;0 0]  Multiplication=Matrix(K*u) (u vector)
  Gain7 : Gain  Gain=Tau_GP  Multiplication=Matrix(K*u) (u vector)
  Gain8 : Gain  Gain=-Tau_GP'  Multiplication=Matrix(K*u) (u vector)
  Gain9 : Gain  Gain=Tau_GP  Multiplication=Matrix(K*u) (u vector)
  Mux : Mux  Inputs=[3 3]
  Omega : RCTblocks/Uncertain State Space  Tag=USS  USystem=uss(Omega*eye(3))  UValue=[]  X0=[]  uX0=[]
  Sum : Sum  Inputs=|++
  Terminator : Terminator
  Terminator1 : Terminator
  W_body/. : Outport  VectorParamsAs1DForOutWhenUnconnected=off
  wires:
  Gain9/1 -> Demux/1
  Mux/1 -> Gain8/1
  Gain8/1 -> W_body/./1
  Omega/1 -> Sum/2
  Gain6/1 -> Omega/1
  Gain5/1 -> Gain6/1
  Sum/1 -> Gain2/1
  Gain4/1 -> Sum/1
  Gain1/1 -> Gain4/1
  Demux/2 -> Gain1/1
  Demux/1 -> Gain3/1
  Gain2/1 -> Mux/2
  Gain3/1 -> Mux/1
  m/1 -> Demux2/1
  Demux2/1 -> Gain9/1
  Demux2/2 -> Gain7/1
  Demux2/3 -> Terminator/1
  Gain7/1 -> Demux3/1
  Demux3/1 -> Terminator1/1
  Demux3/2 -> Gain10/1
  Gain10/1 -> Gain5/1

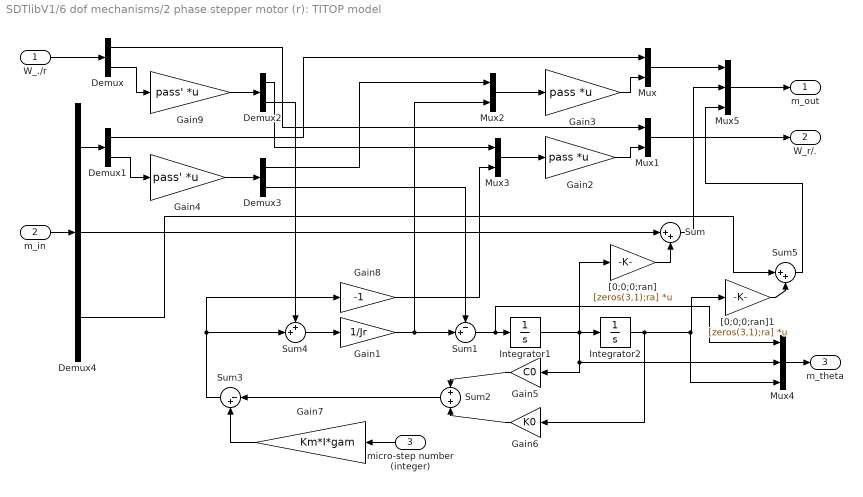
== system SDTlibV1/6 dof mechanisms/2 phase stepper motor (r): TITOP model ==
  W_./r : Inport  PortDimensions=6
  m_in : Inport  Port=2  PortDimensions=18
  micro-step number (integer) : Inport  Port=3  PortDimensions=1
  Demux : Demux  Outputs=[3 3]
  Demux1 : Demux  Outputs=[3 3]
  Demux2 : Demux  Outputs=[2 1]
  Demux3 : Demux  Outputs=[2 1]
  Demux4 : Demux  Outputs=[6 6 6]
  Gain1 : Gain  Gain=1/Jr
  Gain2 : Gain  Gain=pass  Multiplication=Matrix(K*u) (u vector)
  Gain3 : Gain  Gain=pass  Multiplication=Matrix(K*u) (u vector)
  Gain4 : Gain  Gain=pass'  Multiplication=Matrix(K*u) (u vector)
  Gain5 : Gain  Gain=C0
  Gain6 : Gain  Gain=K0
  Gain7 : Gain  Gain=Km*I*gam
  Gain8 : Gain  Gain=-1
  Gain9 : Gain  Gain=pass'  Multiplication=Matrix(K*u) (u vector)
  Integrator1 : Integrator
  Integrator2 : Integrator
  Mux : Mux  Inputs=[3 3]
  Mux1 : Mux  Inputs=[3 3]
  Mux2 : Mux  Inputs=[2 1]
  Mux3 : Mux  Inputs=[2 1]
  Mux4 : Mux  Inputs=3
  Mux5 : Mux  Inputs=[6 6 6]
  Sum : Sum  Inputs=|++
  Sum1 : Sum  Inputs=-+|
  Sum2 : Sum
  Sum3 : Sum  Inputs=|-+
  Sum4 : Sum  Inputs=++|
  Sum5 : Sum  Inputs=|++
  "[0;0;0;ran]" : Gain  Gain=[zeros(3,1);ra]  Multiplication=Matrix(K*u) (u vector)
  "[0;0;0;ran]1" : Gain  Gain=[zeros(3,1);ra]  Multiplication=Matrix(K*u) (u vector)
  m_out : Outport
  W_r/. : Outport  Port=2
  m_theta : Outport  Port=3
  wires:
  Mux1/1 -> W_r/./1
  Demux1/1 -> Mux/1
  Sum3/1 -> Sum4/2, Gain8/1
  Demux/1 -> Mux1/1
  micro-step number (integer)/1 -> Gain7/1
  Gain2/1 -> Mux1/2
  Sum1/1 -> Mux4/1, Integrator1/1
  Demux/2 -> Gain9/1
  Gain1/1 -> Mux2/2, Sum1/2
  Sum2/1 -> Sum3/1
  Integrator1/1 -> "[0;0;0;ran]"/1, Integrator2/1, Gain5/1, Mux4/2
  Sum4/1 -> Gain1/1
  W_./r/1 -> Demux/1
  Gain5/1 -> Sum2/1
  Gain7/1 -> Sum3/2
  Gain6/1 -> Sum2/2
  Gain3/1 -> Mux/2
  Demux3/2 -> Sum1/1
  Gain9/1 -> Demux2/1
  Demux2/2 -> Sum4/1
  Mux2/1 -> Gain3/1
  Demux1/2 -> Gain4/1
  Gain4/1 -> Demux3/1
  Mux3/1 -> Gain2/1
  Gain8/1 -> Mux3/2
  Demux2/1 -> Mux3/1
  Demux3/1 -> Mux2/1
  Demux4/1 -> Demux1/1
  Demux4/2 -> Sum/1
  m_in/1 -> Demux4/1
  Mux/1 -> Mux5/1
  Mux5/1 -> m_out/1
  "[0;0;0;ran]"/1 -> Sum/2
  Sum/1 -> Mux5/2
  "[0;0;0;ran]1"/1 -> Sum5/2
  Integrator2/1 -> Gain6/1, Mux4/3, "[0;0;0;ran]1"/1
  Demux4/3 -> Sum5/1
  Sum5/1 -> Mux5/3
  Mux4/1 -> m_theta/1
